simulink model "ITL_Controle_Adaptativo"  (R2015a)
settings: Solver=ode45  StartTime=0.0  StopTime=10.0  RelTol=1e-3
settings Model: Creator=user  LastModifiedBy=user

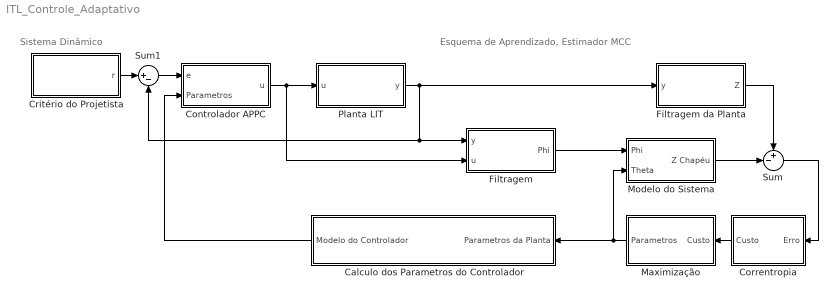
== system ITL_Controle_Adaptativo ==
  note: Sistema Dinâmico
  note: Esquema de Aprendizado, Estimador MCC
  Calculo dos Parametros do Controlador : Subsystem
  Controlador APPC : Subsystem
  Correntropia : Subsystem
  Critério do Projetista : Subsystem
  Filtragem : Subsystem
  Filtragem da Planta : Subsystem
  Maximização : Subsystem
  Modelo do Sistema : Subsystem
  Planta LIT : Subsystem
  Sum : Sum  Inputs=+-|
  Sum1 : Sum  Inputs=|+-
  wires:
  Modelo do Sistema/1(Z Chapéu) -> Sum/2
  Sum/1 -> Correntropia/1(Erro)
  Correntropia/1(Custo) -> Maximização/1(Custo)
  Maximização/1(Parametros) -> Calculo dos Parametros do Controlador/1(Parametros da Planta), Modelo do Sistema/2(Theta)
  Filtragem/1(Phi) -> Modelo do Sistema/1(Phi)
  Filtragem da Planta/1(Z) -> Sum/1
  Controlador APPC/1(u) -> Planta LIT/1(u), Filtragem/2(u)
  Sum1/1 -> Controlador APPC/1(e)
  Critério do Projetista/1(r) -> Sum1/1
  Planta LIT/1(y) -> Filtragem da Planta/1(y), Sum1/2, Filtragem/1(y)
  Calculo dos Parametros do Controlador/1(Modelo do Controlador) -> Controlador APPC/2(Parametros)

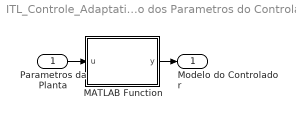
== system ITL_Controle_Adaptativo/Calculo dos Parametros do Controlador ==
  Parametros da Planta : Inport
  MATLAB Function : MATLAB Function  TreatAsAtomicUnit=on
  Modelo do Controlador : Outport
  wires:
  MATLAB Function/1(y) -> Modelo do Controlador/1
  Parametros da Planta/1 -> MATLAB Function/1(u)

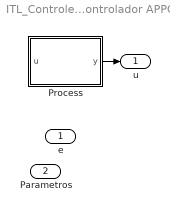
== system ITL_Controle_Adaptativo/Controlador APPC ==
  e : Inport
  Parametros : Inport  Port=2
  Process : MATLAB Function  TreatAsAtomicUnit=on
  u : Outport
  wires:
  Process/1(y) -> u/1

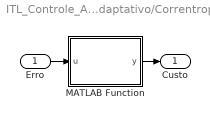
== system ITL_Controle_Adaptativo/Correntropia ==
  Erro : Inport
  MATLAB Function : MATLAB Function  TreatAsAtomicUnit=on
  Custo : Outport
  wires:
  Erro/1 -> MATLAB Function/1(u)
  MATLAB Function/1(y) -> Custo/1

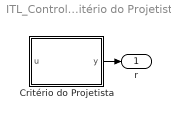
== system ITL_Controle_Adaptativo/Critério do Projetista ==
  Critério do Projetista : MATLAB Function  TreatAsAtomicUnit=on
  r : Outport
  wires:
  Critério do Projetista/1(y) -> r/1

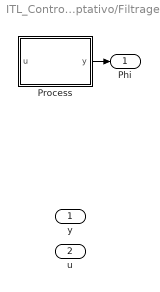
== system ITL_Controle_Adaptativo/Filtragem ==
  y : Inport
  u : Inport  Port=2
  Process : MATLAB Function  TreatAsAtomicUnit=on
  Phi : Outport
  wires:
  Process/1(y) -> Phi/1

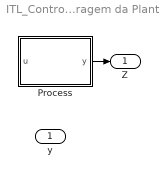
== system ITL_Controle_Adaptativo/Filtragem da Planta ==
  y : Inport
  Process : MATLAB Function  TreatAsAtomicUnit=on
  Z : Outport
  wires:
  Process/1(y) -> Z/1

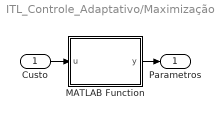
== system ITL_Controle_Adaptativo/Maximização ==
  Custo : Inport
  MATLAB Function : MATLAB Function  TreatAsAtomicUnit=on
  Parametros : Outport
  wires:
  Custo/1 -> MATLAB Function/1(u)
  MATLAB Function/1(y) -> Parametros/1

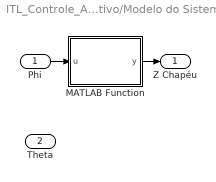
== system ITL_Controle_Adaptativo/Modelo do Sistema ==
  Phi : Inport
  Theta : Inport  Port=2
  MATLAB Function : MATLAB Function  TreatAsAtomicUnit=on
  Z Chapéu : Outport
  wires:
  Phi/1 -> MATLAB Function/1(u)
  MATLAB Function/1(y) -> Z Chapéu/1

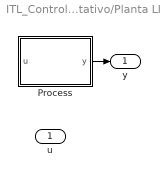
== system ITL_Controle_Adaptativo/Planta LIT ==
  u : Inport
  Process : MATLAB Function  TreatAsAtomicUnit=on
  y : Outport
  wires:
  Process/1(y) -> y/1

== matlab function ITL_Controle_Adaptativo/Correntropia/MATLAB Function ==
  data: u input; y output
function y = fcn(u)
%#codegen

y = u;

== matlab function ITL_Controle_Adaptativo/Modelo do Sistema/MATLAB Function ==
  data: u input; y output
function y = fcn(u)
%#codegen

y = u;

== matlab function ITL_Controle_Adaptativo/Maximização/MATLAB Function ==
  data: u input; y output
function y = fcn(u)
%#codegen

y = u;

== matlab function ITL_Controle_Adaptativo/Filtragem/Process ==
  data: u input; y output
function y = fcn(u)
%#codegen

y = u;

== matlab function ITL_Controle_Adaptativo/Filtragem da Planta/Process ==
  data: u input; y output
function y = fcn(u)
%#codegen

y = u;

== matlab function ITL_Controle_Adaptativo/Planta LIT/Process ==
  data: u input; y output
function y = fcn(u)
%#codegen

y = u;

== matlab function ITL_Controle_Adaptativo/Controlador APPC/Process ==
  data: u input; y output
function y = fcn(u)
%#codegen

y = u;

== matlab function ITL_Controle_Adaptativo/Critério do Projetista/Critério do Projetista ==
  data: u input; y output
function y = fcn(u)
%#codegen

y = u;

== matlab function ITL_Controle_Adaptativo/Calculo dos Parametros do Controlador/MATLAB Function ==
  data: u input; y output
function y = fcn(u)
%#codegen

y = u;
